simulink subsystem "lift_compoenent"  (R2024b)
settings: Solver=VariableStepAuto  StartTime=0.0  StopTime=10.0  RelTol=1e-3
undefined symbols (not defined in the file or in its folder): Ar, OR_cg, sim_time
settings Model: Creator=joedo  LastModifiedBy=finnb

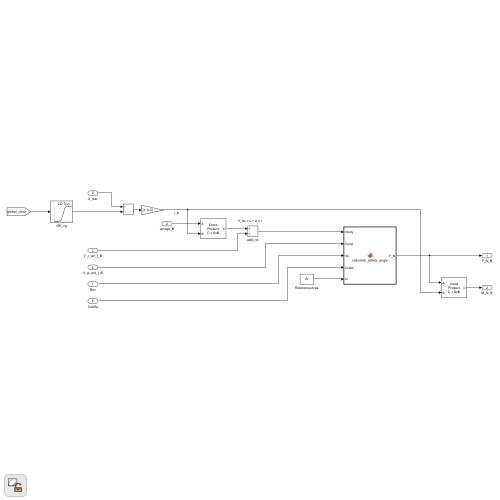
[thumbnail: Simulink's stored preview of the top-level diagram]
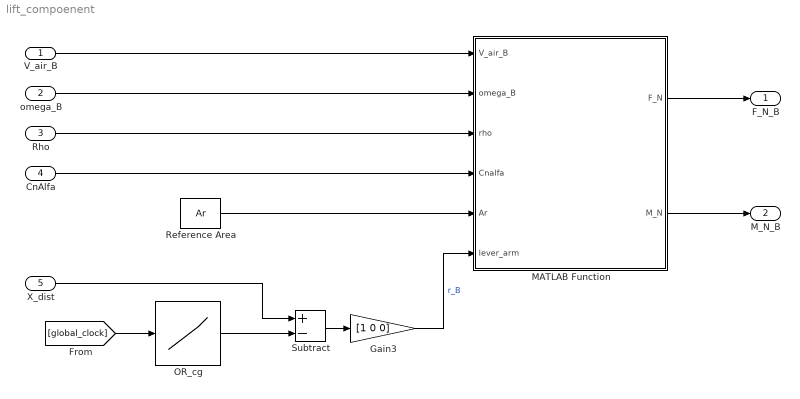
== system lift_compoenent ==
  "V_air_B " : Inport
  omega_B : Inport  Port=2
  Rho : Inport  Port=3
  CnAlfa : Inport  Port=4
  X_dist : Inport  Port=5
  Gain3 : Gain  Gain=[1 0 0]
  MATLAB Function : MATLAB Function  TreatAsAtomicUnit=on
  OR_cg : Lookup_n-D  NumberOfTableDimensions=1  BreakpointsForDimension1=sim_time  Table=OR_cg  InternalRulePriority=Speed  RndMeth=Simplest
  Reference Area : Constant  Value=Ar
  Subtract : Sum  Inputs=+-
  F_N_B : Outport  VectorParamsAs1DForOutWhenUnconnected=off
  M_N_B : Outport  Port=2  VectorParamsAs1DForOutWhenUnconnected=off
  wires:
  OR_cg/1 -> Subtract/2
  [global_clock] -> OR_cg/1
  Subtract/1 -> Gain3/1
  X_dist/1 -> Subtract/1
  Reference Area/1 -> MATLAB Function/5(Ar)
  CnAlfa/1 -> MATLAB Function/4(Cnalfa)
  Gain3/1 -> MATLAB Function/6(lever_arm)  "r_B"
  MATLAB Function/2(M_N) -> M_N_B/1
  Rho/1 -> MATLAB Function/3(rho)
  "V_air_B "/1 -> MATLAB Function/1(V_air_B)
  omega_B/1 -> MATLAB Function/2(omega_B)
  MATLAB Function/1(F_N) -> F_N_B/1

== matlab function lift_compoenent/MATLAB Function ==
  data: V_air_B input; omega_B input; rho input; Cnalfa input; Ar input; lever_arm input; F_N output; M_N output
function [F_N, M_N] = calculate_normal_force(V_air_B, omega_B, rho, Cnalfa, Ar, lever_arm)
    % relative velocity
    Vrel = V_air_B + cross(omega_B, lever_arm);
    
    % Body relative velocity magnitude
    Vrel_mag = norm(Vrel);
    VrelMagYZ = norm(Vrel(2:3));
    
    if VrelMagYZ ~= 0 % prevent division by 0
        % Angle of attack and component separation
        attack_angle = asin(VrelMagYZ/Vrel_mag);
        F_N_dir = [0; Vrel(2) / VrelMagYZ; Vrel(3) / VrelMagYZ];
        
        % Calculating total force
        F_N_mag = 0.5 * rho * Vrel_mag^2 * Ar * Cnalfa * attack_angle;
        F_N = F_N_dir * F_N_mag;
    else
        F_N = [0; 0; 0];
    end
    % Total torque
    M_N = cross(F_N, lever_arm);
end
